simulink model "PMSM_global_dyn_sys_NL"  (R2018a)
settings: Solver=FixedStepAuto  StartTime=0.0  StopTime=5  FixedStep=0.0001  RelTol=1e-3
values from neighbouring files (symbols this model uses):
  b_eq = b_m + b_l/r^2    (= 1.5637748692e-05)    [PMSM_AyME.m]    (also in estabilidad_open_loop.m)
  C_t = 1.091    [PMSM_AyME.m]
  J_eq = J_m + J_l/r^2    (= 5.65099476805e-06)    [PMSM_AyME.m]    (also in estabilidad_open_loop.m)
  L_d = 6.6E-3    (= 0.0066)    [PMSM_AyME.m]    (also in estabilidad_open_loop.m)
  L_q = 5.8E-3    (= 0.0058)    [PMSM_AyME.m]    (also in estabilidad_open_loop.m)
  lambda_m = 0.01546    [PMSM_AyME.m]    (also in estabilidad_open_loop.m)
  Lls = 0.8E-3    (= 0.0008)    [PMSM_AyME.m]    (also in estabilidad_open_loop.m)
  Pp = 3    [PMSM_AyME.m]    (also in estabilidad_open_loop.m)
  R_s = 1.02    [PMSM_AyME.m]    (also in estabilidad_open_loop.m)
  R_tsa = 55    [PMSM_AyME.m]
  Tl_eq = Tl/r    (= 0.00499521477515)    [PMSM_AyME.m]    (also in estabilidad_open_loop.m)
undefined symbols (not defined in the file or in its folder): sigbuilder_block
libraries: dspsigops x3, peTransforms x1
settings Model: Creator=gino  LastModifiedBy=gino

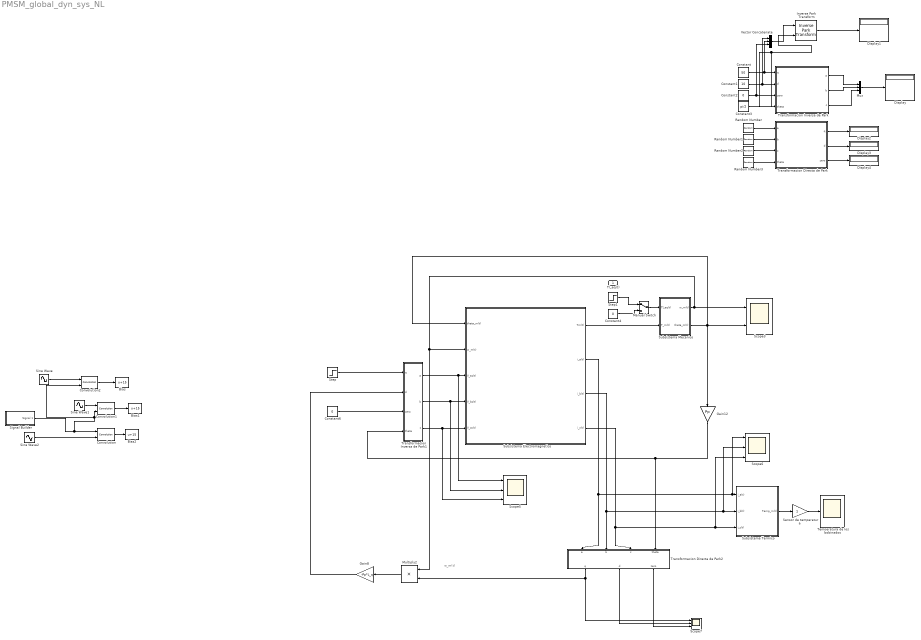
== system PMSM_global_dyn_sys_NL ==
  note: w_m(t)
  Tl_eq(t) : Inport
  Bias : Bias  Bias=15
  Bias1 : Bias  Bias=15
  Bias2 : Bias  Bias=15
  Constant : Constant  Value=50
  Constant1 : Constant  Value=10
  Constant2 : Constant  Value=0
  Constant3 : Constant  Value=pi/2
  Constant4 : Constant  Value=0
  Constant6 : Constant  Value=0
  Convolution : dspsigops/Convolution  domain=Time  roundingMode=Floor  overflowMode=off  outputDataTypeStr=Inherit: Same as accumulator  outputMin=[]  outputMax=[]  outputLastDataTypeStr=Inherit: Same as accumulator
      settings: SourceProductName=DSP System Toolbox  SourceProductBaseCode=DS
  Convolution1 : dspsigops/Convolution  domain=Time  roundingMode=Floor  overflowMode=off  outputDataTypeStr=Inherit: Same as accumulator  outputMin=[]  outputMax=[]  outputLastDataTypeStr=Inherit: Same as accumulator
      settings: SourceProductName=DSP System Toolbox  SourceProductBaseCode=DS
  Convolution2 : dspsigops/Convolution  domain=Time  roundingMode=Floor  overflowMode=off  outputDataTypeStr=Inherit: Same as accumulator  outputMin=[]  outputMax=[]  outputLastDataTypeStr=Inherit: Same as accumulator
      settings: SourceProductName=DSP System Toolbox  SourceProductBaseCode=DS
  Display{,1..4} (5 alike) : Display
  Gain12 : Gain  Gain=Pp
  Gain8 : Gain  Gain=-Pp*L_q
  Inverse Park Transform : peTransforms/Inverse Park Transform  AxisAlignment=Q-axis  PowerInvariant=off
  Manual Switch : ManualSwitch
  Multiply2 : Product
  Mux : Mux  Inputs=3
  Random Number{,1..3} (4 alike) : RandomNumber  SampleTime=0.1
  Scope3 : Scope  NumInputPorts=2
  Scope5 : Scope  NumInputPorts=3
  Scope6 : Scope  NumInputPorts=3
  Scope7 : Scope  NumInputPorts=3
  Sensor de temperatura : Gain
  Signal Builder : Subsystem  Tag=STV Subsys  LoadFcn=sigbuilder_block('load');  StartFcn=sigbuilder_block('start');  StopFcn=sigbuilder_block('stop');  ClipboardFcn=sigbuilder_block('clipboard');  mask(Sigbuilder block){tuvar=[0:10]}
      mask help: Simulink:masks:SigbuilderBlock_MD
      mask init:
      | if ~strcmp(get_param(bdroot(gcbh),'SimulationStatus'),'stopped') tuvar = sigbuilder_block('maskInit'); end
      settings: CopyFcn=sigbuilder_block('copy');  DeleteFcn=sigbuilder_block('delete');  ModelCloseFcn=sigbuilder_block('modelClose');  PreSaveFcn=sigbuilder_block('preSave');  PauseFcn=sigbuilder_block('pause');  ContinueFcn=sigbuilder_block('continue');  NameChangeFcn=sigbuilder_block('namechange');  OpenFcn=sigbuilder_block('open',[242.25 102.75 550.5 357 ]);  CloseFcn=sigbuilder_block('close');
      mask Display: plot(0, 0, 100, 100,[2, 2, 32, 32, 2], [68, 8, 8, 68, 68],[32, 2], [38, 38], [32, 19, 2],[53, 60, 44], [32, 17, 17, 2],[16, 16, 31, 31]);txt = getActiveGroup(gcbh);text(2, 100, txt,'verticalAlignment', 'top');
  Sine Wave : Sin  Amplitude=30  Frequency=300*2*pi  SampleTime=0
  Sine Wave1 : Sin  Amplitude=30  Frequency=300*2*pi  Phase=2*pi/3  SampleTime=0
  Sine Wave2 : Sin  Amplitude=30  Frequency=300*2*pi  Phase=4*pi/3  SampleTime=0
  Step : Step  Time=0.1  After=19.596  SampleTime=0
  Step1 : Step  Time=0.3  After=Tl_eq  SampleTime=0
  Subsistema Mecanico : Subsystem
  Subsistema Electromagnetico : Subsystem
  Subsistema Termico : Subsystem
  Temperatura de los bobinados : Scope
  Transformacion Directa de Park : MATLAB Function  TreatAsAtomicUnit=on
  Transformacion Directa de Park2 : MATLAB Function  TreatAsAtomicUnit=on
  Transformacion Inversa de Park : MATLAB Function  TreatAsAtomicUnit=on
  Transformacion Inversa de Park1 : MATLAB Function  TreatAsAtomicUnit=on
  Vector Concatenate : Concatenate  NumInputs=3
  wires:
  Subsistema Electromagnetico/1(Tm(t)) -> Subsistema Mecanico/2(T_m(t))
  Constant3/1 -> Inverse Park Transform/2, Transformacion Inversa de Park/4(theta)
  Constant2/1 -> Vector Concatenate/3, Transformacion Inversa de Park/3(zero)
  Constant1/1 -> Vector Concatenate/1, Transformacion Inversa de Park/2(d)
  Constant/1 -> Vector Concatenate/2, Transformacion Inversa de Park/1(q)
  Transformacion Inversa de Park/2(b) -> Mux/2
  Transformacion Inversa de Park/1(a) -> Mux/1
  Transformacion Inversa de Park/3(c) -> Mux/3
  Mux/1 -> Display/1
  Vector Concatenate/1 -> Inverse Park Transform/1
  Inverse Park Transform/1 -> Display1/1
  Subsistema Mecanico/1(w_m(t)) -> Scope3/1, Subsistema Electromagnetico/2(w_m(t)), Multiply2/1
  Subsistema Mecanico/2(theta_m(t)) -> Subsistema Electromagnetico/1("theta_m(t) "), Gain12/1, Scope3/2
  Manual Switch/1 -> Subsistema Mecanico/1(Tl_eq(t))
  Constant4/1 -> Manual Switch/2
  Subsistema Electromagnetico/2(i_a(t)) -> Scope6/1, Subsistema Termico/1(i_a(t)), Transformacion Directa de Park2/1(a)
  Subsistema Electromagnetico/3(i_b(t)) -> Subsistema Termico/2(i_b(t)), Scope6/2, Transformacion Directa de Park2/2(b)
  Subsistema Electromagnetico/4(i_c(t)) -> Subsistema Termico/3(i_c(t)), Scope6/3, Transformacion Directa de Park2/3(c)
  Convolution1/1 -> Bias1/1
  Signal Builder/1(Signal 1) -> Convolution/1, Convolution1/2, Convolution2/2
  Sine Wave2/1 -> Convolution/2
  Sine Wave1/1 -> Convolution1/1
  Sine Wave/1 -> Convolution2/1
  Convolution/1 -> Bias2/1
  Convolution2/1 -> Bias/1
  Random Number2/1 -> Transformacion Directa de Park/3(c)
  Random Number3/1 -> Transformacion Directa de Park/4(theta)
  Random Number1/1 -> Transformacion Directa de Park/2(b)
  Random Number/1 -> Transformacion Directa de Park/1(a)
  Transformacion Directa de Park/3(zero) -> Display4/1
  Transformacion Directa de Park/2(d) -> Display3/1
  Transformacion Directa de Park/1(q) -> Display2/1
  Subsistema Termico/1(Temp_m(t)) -> Sensor de temperatura/1
  Transformacion Inversa de Park1/1(a) -> Subsistema Electromagnetico/3(V_as(t)), Scope5/1
  Transformacion Inversa de Park1/2(b) -> Subsistema Electromagnetico/4(V_bs(t)), Scope5/2
  Transformacion Inversa de Park1/3(c) -> Subsistema Electromagnetico/5(V_cs(t)), Scope5/3
  Step/1 -> Transformacion Inversa de Park1/1(q)
  Gain12/1 -> Transformacion Directa de Park2/4(theta), Transformacion Inversa de Park1/4(theta)
  Transformacion Directa de Park2/1(q) -> Multiply2/2, Scope7/1
  Multiply2/1 -> Gain8/1
  Gain8/1 -> Transformacion Inversa de Park1/2(d)
  Constant6/1 -> Transformacion Inversa de Park1/3(zero)
  Step1/1 -> Manual Switch/1
  Sensor de temperatura/1 -> Temperatura de los bobinados/1
  Transformacion Directa de Park2/2(d) -> Scope7/2
  Transformacion Directa de Park2/3(zero) -> Scope7/3

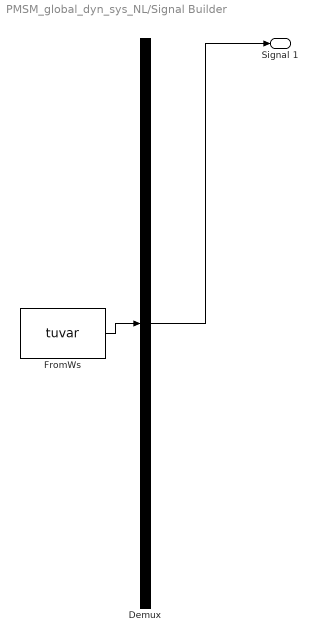
== system PMSM_global_dyn_sys_NL/Signal Builder ==
  Demux : Demux  Tag=STV Demux  Outputs=1
  FromWs : FromWorkspace  Tag=STV FromWs  VariableName=tuvar  SampleTime=0
      SigBuilderData=|
      | common.afterFinalStr = 'Extrapolate'
      | common.sampleTime = 0
      | dataSet.timeRange = [0 10]
      | dataSet.name = 'Group 1'
      | sbobj.Groups.Name = 'Group 1'
      | sbobj.Groups.Signals.Name = 'Signal 1'
      | sbobj.Groups.Signals.XData = [0 0.49 10]
      | sbobj.Groups.Signals.YData = [0 1 1]
  Signal 1 : Outport  Tag=STV Outport
  wires:
  Demux/1 -> Signal 1/1
  FromWs/1 -> Demux/1

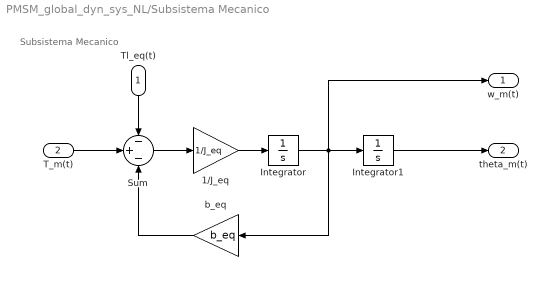
== system PMSM_global_dyn_sys_NL/Subsistema Mecanico ==
  note: Subsistema Mecanico
  Tl_eq(t) : Inport
  T_m(t) : Inport  Port=2
  1/J_eq : Gain  Gain=1/J_eq
  Integrator : Integrator
  Integrator1 : Integrator
  Sum : Sum  Inputs=-+-
  b_eq : Gain  Gain=b_eq
  w_m(t) : Outport
  theta_m(t) : Outport  Port=2
  wires:
  1/J_eq/1 -> Integrator/1
  Integrator1/1 -> theta_m(t)/1
  Integrator/1 -> Integrator1/1, w_m(t)/1, b_eq/1
  Sum/1 -> 1/J_eq/1
  Tl_eq(t)/1 -> Sum/1
  b_eq/1 -> Sum/3
  T_m(t)/1 -> Sum/2

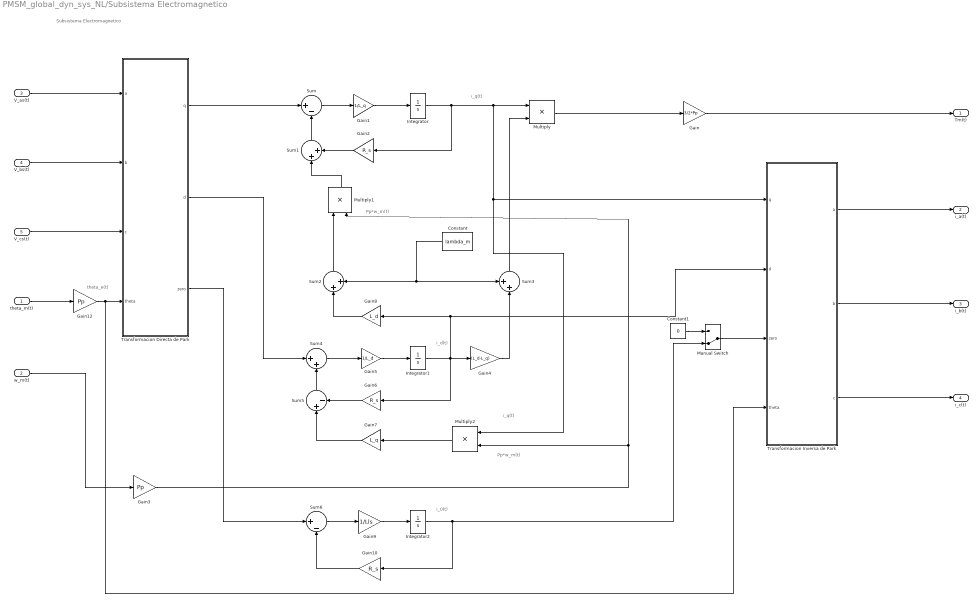
== system PMSM_global_dyn_sys_NL/Subsistema Electromagnetico ==
  note: Subsistema Electromagnetico
  note: theta_e(t)
  note: i_0(t)
  note: Pp*w_m(t)
  note: Pp*w_m(t)
  note: i_q(t)
  note: i_d(t)
  note: i_q(t)
  "theta_m(t) " : Inport
  w_m(t) : Inport  Port=2
  V_as(t) : Inport  Port=3
  V_bs(t) : Inport  Port=4
  V_cs(t) : Inport  Port=5
  Constant : Constant  Value=lambda_m
  Constant1 : Constant  Value=0
  Gain : Gain  Gain=3/2*Pp
  Gain1 : Gain  Gain=1/L_q
  Gain10 : Gain  Gain=R_s
  Gain12 : Gain  Gain=Pp
  Gain2 : Gain  Gain=R_s
  Gain3 : Gain  Gain=Pp
  Gain4 : Gain  Gain=(L_d-L_q)
  Gain5 : Gain  Gain=1/L_d
  Gain6 : Gain  Gain=R_s
  Gain7 : Gain  Gain=L_q
  Gain8 : Gain  Gain=L_d
  Gain9 : Gain  Gain=1/Lls
  Integrator : Integrator
  Integrator1 : Integrator
  Integrator2 : Integrator
  Manual Switch : ManualSwitch  CurrentSetting=0
  Multiply : Product
  Multiply1 : Product
  Multiply2 : Product
  Sum : Sum  Inputs=|+-
  Sum1 : Sum  Inputs=|++
  Sum2 : Sum  Inputs=|++
  Sum3 : Sum  Inputs=++|
  Sum4 : Sum  Inputs=|++
  Sum5 : Sum  Inputs=|+-
  Sum6 : Sum  Inputs=|+-
  Transformacion Directa de Park : MATLAB Function  TreatAsAtomicUnit=on
  Transformacion Inversa de Park : MATLAB Function  TreatAsAtomicUnit=on
  Tm(t) : Outport
  i_a(t) : Outport  Port=2
  i_b(t) : Outport  Port=3
  i_c(t) : Outport  Port=4
  wires:
  Gain/1 -> Tm(t)/1
  Multiply/1 -> Gain/1
  Integrator/1 -> Gain2/1, Transformacion Inversa de Park/1(q), Multiply2/1, Multiply/1
  Gain1/1 -> Integrator/1
  Sum/1 -> Gain1/1
  Sum1/1 -> Sum/2
  Gain2/1 -> Sum1/2
  Multiply1/1 -> Sum1/1
  w_m(t)/1 -> Gain3/1
  Gain3/1 -> Multiply1/2, Multiply2/2
  Sum2/1 -> Multiply1/1
  Sum3/1 -> Multiply/2
  Constant/1 -> Sum3/1, Sum2/2
  Gain4/1 -> Sum3/2
  Integrator1/1 -> Transformacion Inversa de Park/2(d), Gain8/1, Gain4/1, Gain6/1
  Gain5/1 -> Integrator1/1
  Sum4/1 -> Gain5/1
  Gain6/1 -> Sum5/2
  Gain7/1 -> Sum5/1
  Multiply2/1 -> Gain7/1
  Gain8/1 -> Sum2/1
  Sum5/1 -> Sum4/2
  Transformacion Directa de Park/1(q) -> Sum/1
  Transformacion Directa de Park/2(d) -> Sum4/1
  Gain9/1 -> Integrator2/1
  Sum6/1 -> Gain9/1
  Gain10/1 -> Sum6/2
  Integrator2/1 -> Manual Switch/2, Gain10/1
  Transformacion Directa de Park/3(zero) -> Sum6/1
  "theta_m(t) "/1 -> Gain12/1
  Gain12/1 -> Transformacion Directa de Park/4(theta), Transformacion Inversa de Park/4(theta)
  V_as(t)/1 -> Transformacion Directa de Park/1(a)
  V_bs(t)/1 -> Transformacion Directa de Park/2(b)
  V_cs(t)/1 -> Transformacion Directa de Park/3(c)
  Manual Switch/1 -> Transformacion Inversa de Park/3(zero)
  Constant1/1 -> Manual Switch/1
  Transformacion Inversa de Park/1(a) -> i_a(t)/1
  Transformacion Inversa de Park/2(b) -> i_b(t)/1
  Transformacion Inversa de Park/3(c) -> i_c(t)/1

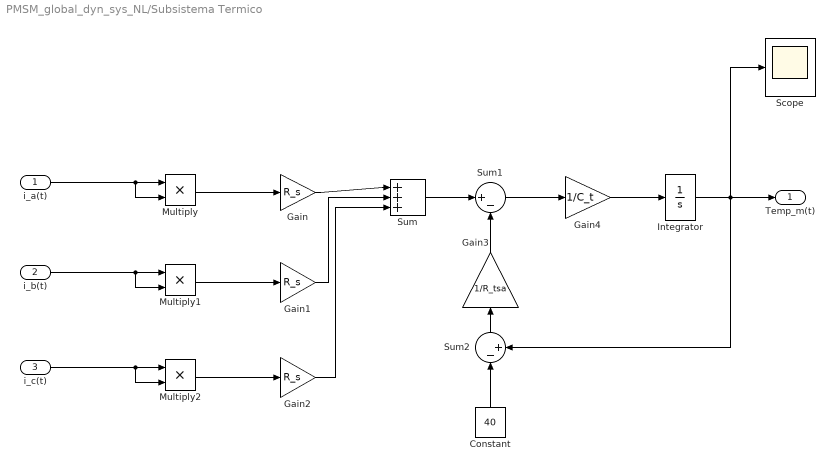
== system PMSM_global_dyn_sys_NL/Subsistema Termico ==
  i_a(t) : Inport
  i_b(t) : Inport  Port=2
  i_c(t) : Inport  Port=3
  Constant : Constant  Value=40
  Gain : Gain  Gain=R_s
  Gain1 : Gain  Gain=R_s
  Gain2 : Gain  Gain=R_s
  Gain3 : Gain  Gain=1/R_tsa
  Gain4 : Gain  Gain=1/C_t
  Integrator : Integrator  InitialCondition=40
  Multiply : Product
  Multiply1 : Product
  Multiply2 : Product
  Scope : Scope
  Sum : Sum  Inputs=|+++
  Sum1 : Sum  Inputs=|+-
  Sum2 : Sum  Inputs=|-+
  Temp_m(t) : Outport
  wires:
  i_a(t)/1 -> Multiply/1, Multiply/2
  i_b(t)/1 -> Multiply1/2, Multiply1/1
  i_c(t)/1 -> Multiply2/2, Multiply2/1
  Multiply/1 -> Gain/1
  Multiply1/1 -> Gain1/1
  Multiply2/1 -> Gain2/1
  Gain1/1 -> Sum/2
  Gain/1 -> Sum/1
  Gain2/1 -> Sum/3
  Sum/1 -> Sum1/1
  Gain3/1 -> Sum1/2
  Sum2/1 -> Gain3/1
  Constant/1 -> Sum2/1
  Sum1/1 -> Gain4/1
  Gain4/1 -> Integrator/1
  Integrator/1 -> Sum2/2, Temp_m(t)/1, Scope/1

== matlab function PMSM_global_dyn_sys_NL/Transformacion Inversa de Park ==
  data: q input; a output; d input; zero input; theta input; b output; c output
function [a, b, c] = inverse_park_transformation(q, d, zero, theta)
%Transformación inversa de Park
 
abc = [cos(theta)               sin(theta)              1
        cos(theta - 2*pi/3)     sin(theta - 2*pi/3)     1
        cos(theta + 2*pi/3)     sin(theta + 2*pi/3)     1] ...
    *   [q
        d
        zero];

a = abc(1);
b = abc(2);
c = abc(3);

end

== matlab function PMSM_global_dyn_sys_NL/Transformacion Directa de Park ==
  data: a input; q output; b input; c input; theta input; d output; zero output
function [q, d, zero] = park_transformation(a, b, c, theta)
%Transformación directa de Park
 
qdz = 2/3 * [cos(theta)     cos(theta - 2*pi/3)     cos(theta + 2*pi/3)
                    sin(theta)      sin(theta - 2*pi/3)     sin(theta + 2*pi/3)
                    1/2             1/2                     1/2] ...
                *   [a
                    b 
                    c];

q = qdz(1);
d = qdz(2);
zero = qdz(3);

end

== matlab function PMSM_global_dyn_sys_NL/Subsistema Electromagnetico/Transformacion Directa de Park ==
  data: a input; q output; b input; c input; theta input; d output; zero output
function [q, d, zero] = park_transformation(a, b, c, theta)
%Transformación directa de Park
 
qdz = 2/3 * [cos(theta)     cos(theta - 2*pi/3)     cos(theta + 2*pi/3)
                    sin(theta)      sin(theta - 2*pi/3)     sin(theta + 2*pi/3)
                    1/2             1/2                     1/2] ...
                *   [a
                    b 
                    c];

q = qdz(1);
d = qdz(2);
zero = qdz(3);

end

== matlab function PMSM_global_dyn_sys_NL/Subsistema Electromagnetico/Transformacion Inversa de Park ==
  data: q input; a output; d input; zero input; theta input; b output; c output
function [a, b, c] = inverse_park_transformation(q, d, zero, theta)
%Transformación inversa de Park
 
abc = [cos(theta)               sin(theta)              1
        cos(theta - 2*pi/3)     sin(theta - 2*pi/3)     1
        cos(theta + 2*pi/3)     sin(theta + 2*pi/3)     1] ...
    *   [q
        d
        zero];

a = abc(1);
b = abc(2);
c = abc(3);

end

== matlab function PMSM_global_dyn_sys_NL/Transformacion Inversa de Park1 ==
  data: q input; a output; d input; zero input; theta input; b output; c output
function [a, b, c] = inverse_park_transformation(q, d, zero, theta)
%Transformación inversa de Park
 
abc = [cos(theta)               sin(theta)              1
        cos(theta - 2*pi/3)     sin(theta - 2*pi/3)     1
        cos(theta + 2*pi/3)     sin(theta + 2*pi/3)     1] ...
    *   [q
        d
        zero];

a = abc(1);
b = abc(2);
c = abc(3);

end

== matlab function PMSM_global_dyn_sys_NL/Transformacion Directa de Park2 ==
  data: a input; q output; b input; c input; theta input; d output; zero output
function [q, d, zero] = park_transformation(a, b, c, theta)
%Transformación directa de Park
 
qdz = 2/3 * [cos(theta)     cos(theta - 2*pi/3)     cos(theta + 2*pi/3)
                    sin(theta)      sin(theta - 2*pi/3)     sin(theta + 2*pi/3)
                    1/2             1/2                     1/2] ...
                *   [a
                    b 
                    c];

q = qdz(1);
d = qdz(2);
zero = qdz(3);

end
